simulink model "Example_9_Regulation_Mass_Spring_Damper_System_Mdl"  (Simulink 7.8)
settings: Solver=ode45  StartTime=0.0  StopTime=30  RelTol=1e-3
values from neighbouring files (symbols this model uses):
  A = sys.a    [Example_2_Control.m]    (also in Example_2_Discretization.m; Example_2_Disturbance_Estimation.m; Example_2_Integral_Control.m; Example_2_Prediction_Observer.m)
  B = sys.b    [Example_2_Control.m]    (also in Example_2_Discretization.m; Example_2_Disturbance_Estimation.m; Example_2_Integral_Control.m; Example_2_Prediction_Observer.m)
  ctrl = MPCController(sys,5)    [Example_9_Code_Generation.m]    (also in Example_9_Regulation.m = MPCController(sys,N); Example_9_Regulation_Mass_Spring_Damper_System.m = MPCController(sys,N); Example_9_Tracking.m; Example_9_Tracking_Delta_Input_Formulation.m)
  Ts = 1    [Example_9_Code_Generation.m]    (also in Example_9_Modeling_Simulation.m; Example_9_Regulation.m; Example_9_Tracking.m; Example_9_Tracking_Delta_Input_Formulation.m)
settings Model: Creator=d_goerges  LastModifiedBy=d_goerges
settings DataIOCC: SignalLoggingSaveFormat=Dataset
settings OptimizationCC: ExpressionDepthLimit=128
settings DebuggingCC: UnderspecifiedInitializationDetection=Simplified  MergeDetectMultiDrivingBlocksExec=error  SolverPrmCheckMsg=none  FrameProcessingCompatibilityMsg=error  StateNameClashWarn=none
settings CodeAppCC: CustomSymbolStrType=$N$R$M_T
settings GRTTargetCC: TargetFunctionLibrary=C89/C90 (ANSI)

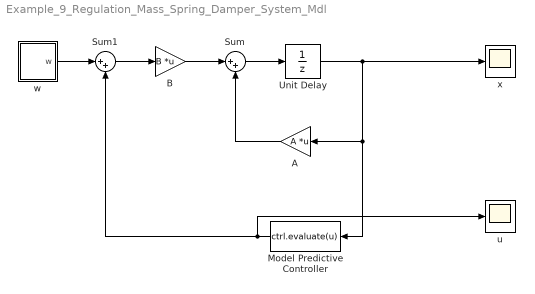
== system Example_9_Regulation_Mass_Spring_Damper_System_Mdl ==
  A : Gain  Gain=A  Multiplication=Matrix(K*u)
  B : Gain  Gain=B  Multiplication=Matrix(K*u)
  Model Predictive Controller : MATLABFcn  MATLABFcn=ctrl.evaluate(u)
  Sum : Sum  Inputs=|++
  Sum1 : Sum  Inputs=|++
  Unit Delay : UnitDelay  X0=[0; 0]  SampleTime=Ts
  u : Scope
      settings: SaveName=ScopeData2
  w : Subsystem
  x : Scope
  wires:
  Unit Delay/1 -> Model Predictive Controller/1, A/1, x/1
  Sum/1 -> Unit Delay/1
  A/1 -> Sum/2
  B/1 -> Sum/1
  Sum1/1 -> B/1
  Model Predictive Controller/1 -> u/1, Sum1/2
  w/1(w) -> Sum1/1

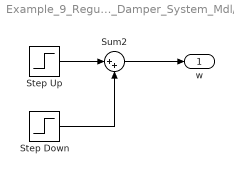
== system Example_9_Regulation_Mass_Spring_Damper_System_Mdl/w ==
  Step Down : Step  Time=3  After=-0.1  SampleTime=0
  Step Up : Step  Time=2  After=0.1  SampleTime=0
  Sum2 : Sum  Inputs=|++
  w : Outport
  wires:
  Sum2/1 -> w/1
  Step Up/1 -> Sum2/1
  Step Down/1 -> Sum2/2
